simulink model "Sim_Ex33"  (R2017a)
settings: Solver=VariableStepAuto  StartTime=0.0  StopTime=Stop_Time  MaxStep=Ts  RelTol=1e-3
values from neighbouring files (symbols this model uses):
  Stop_Time = 0.12    [A_Ex33.m]
  Ts = 1/Fs    (= 5e-05)    [A_Ex33.m]
undefined symbols (not defined in the file or in its folder): DiscIntNeverNeededParam, Grid, PLL
libraries: simulink x3
settings Model: Creator=Joonhee  LastModifiedBy=Joonhee
settings SolverCC: MaxConsecutiveMinStep=1000

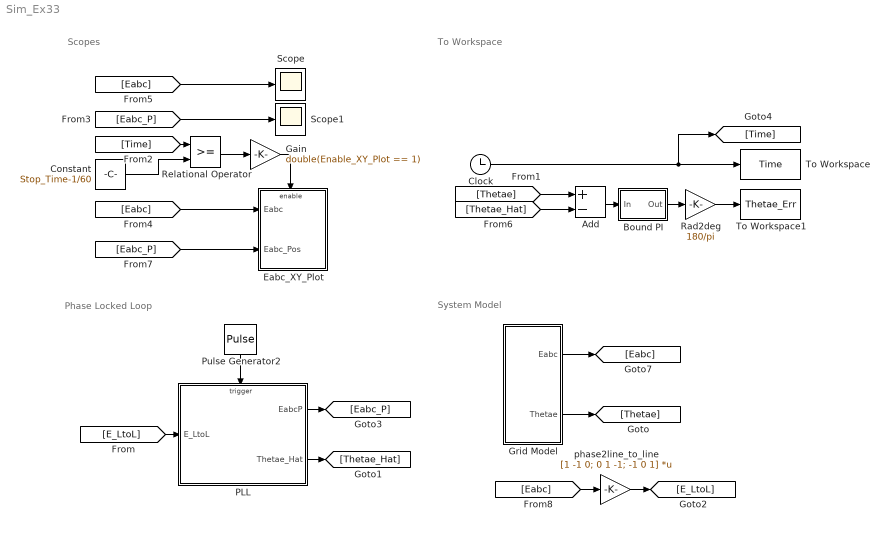
== system Sim_Ex33 ==
  note: System Model
  note: Phase Locked Loop
  note: Scopes
  note: To Workspace
  Add : Sum  Inputs=+-
  Bound PI : Subsystem
  Clock : Clock
  Constant : Constant  Value=Stop_Time-1/60
  Eabc_XY_Plot : Subsystem
  Gain : Gain  Gain=double(Enable_XY_Plot == 1)
  Grid Model : Subsystem
  PLL : Subsystem  TreatAsAtomicUnit=on
  Pulse Generator2 : DiscretePulseGenerator  PulseType=Time based  Period=Ts  PulseWidth=50
  Rad2deg : Gain  Gain=180/pi
  Relational Operator : RelationalOperator  OutDataTypeStr=boolean  RndMeth=Simplest
  Scope : Scope
  Scope1 : Scope
  To Workspace : ToWorkspace  VariableName=Time  SampleTime=Ts
  To Workspace1 : ToWorkspace  VariableName=Thetae_Err  SampleTime=Ts
  phase2line_to_line : Gain  Gain=[1 -1 0; 0 1 -1; -1 0 1]  Multiplication=Matrix(K*u)
  wires:
  Pulse Generator2/1 -> PLL/Trigger
  PLL/2(Thetae_Hat) -> [Thetae_Hat]
  PLL/1(EabcP) -> [Eabc_P]
  [E_LtoL] -> PLL/1(E_LtoL)
  Add/1 -> Bound PI/1(In)
  Bound PI/1(Out) -> Rad2deg/1
  [Thetae_Hat] -> Add/2
  Rad2deg/1 -> To Workspace1/1
  [Eabc] -> Scope/1
  [Eabc_P] -> Scope1/1
  [Thetae] -> Add/1
  Clock/1 -> To Workspace/1, [Time]
  Relational Operator/1 -> Gain/1
  [Time] -> Relational Operator/1
  Constant/1 -> Relational Operator/2
  [Eabc] -> Eabc_XY_Plot/1(Eabc)
  [Eabc_P] -> Eabc_XY_Plot/2(Eabc_Pos)
  Gain/1 -> Eabc_XY_Plot/Enable
  phase2line_to_line/1 -> [E_LtoL]
  [Eabc] -> phase2line_to_line/1
  Grid Model/2(Thetae) -> [Thetae]
  Grid Model/1(Eabc) -> [Eabc]

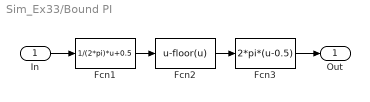
== system Sim_Ex33/Bound PI ==
  In : Inport
  Fcn1 : Fcn  Expr=1/(2*pi)*u+0.5
  Fcn2 : Fcn  Expr=u-floor(u)
  Fcn3 : Fcn  Expr=2*pi*(u-0.5)
  Out : Outport
  wires:
  Fcn1/1 -> Fcn2/1
  Fcn2/1 -> Fcn3/1
  In/1 -> Fcn1/1
  Fcn3/1 -> Out/1

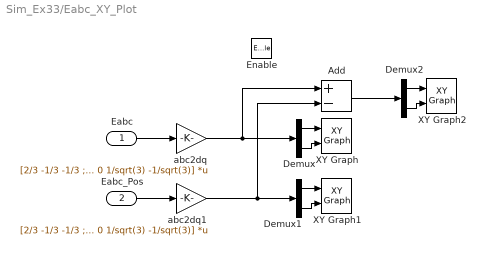
== system Sim_Ex33/Eabc_XY_Plot ==
  Eabc : Inport
  Eabc_Pos : Inport  Port=2
  Enable : EnablePort
  Add : Sum  Inputs=+-
  Demux : Demux  Outputs=2
  Demux1 : Demux  Outputs=2
  Demux2 : Demux  Outputs=2
  XY Graph : simulink/Sinks/XY Graph  xmin=-180  xmax=180  ymin=-180  ymax=180  st=-1
  XY Graph1 : simulink/Sinks/XY Graph  xmin=-180  xmax=180  ymin=-180  ymax=180  st=-1
  XY Graph2 : simulink/Sinks/XY Graph  xmin=-180  xmax=180  ymin=-180  ymax=180  st=-1
  abc2dq : Gain  Gain=[2/3 -1/3 -1/3 ; 0 1/sqrt(3) -1/sqrt(3)]  Multiplication=Matrix(K*u)  SaturateOnIntegerOverflow=on  OutDataTypeStr=Inherit: Same as input  ParamDataTypeStr=Inherit: Same as input
  abc2dq1 : Gain  Gain=[2/3 -1/3 -1/3 ; 0 1/sqrt(3) -1/sqrt(3)]  Multiplication=Matrix(K*u)  SaturateOnIntegerOverflow=on  OutDataTypeStr=Inherit: Same as input  ParamDataTypeStr=Inherit: Same as input
  wires:
  Demux/1 -> XY Graph/1
  Eabc/1 -> abc2dq/1
  Demux1/2 -> XY Graph1/2
  Demux1/1 -> XY Graph1/1
  abc2dq1/1 -> Add/2, Demux1/1
  Demux/2 -> XY Graph/2
  Eabc_Pos/1 -> abc2dq1/1
  abc2dq/1 -> Add/1, Demux/1
  Demux2/2 -> XY Graph2/2
  Demux2/1 -> XY Graph2/1
  Add/1 -> Demux2/1

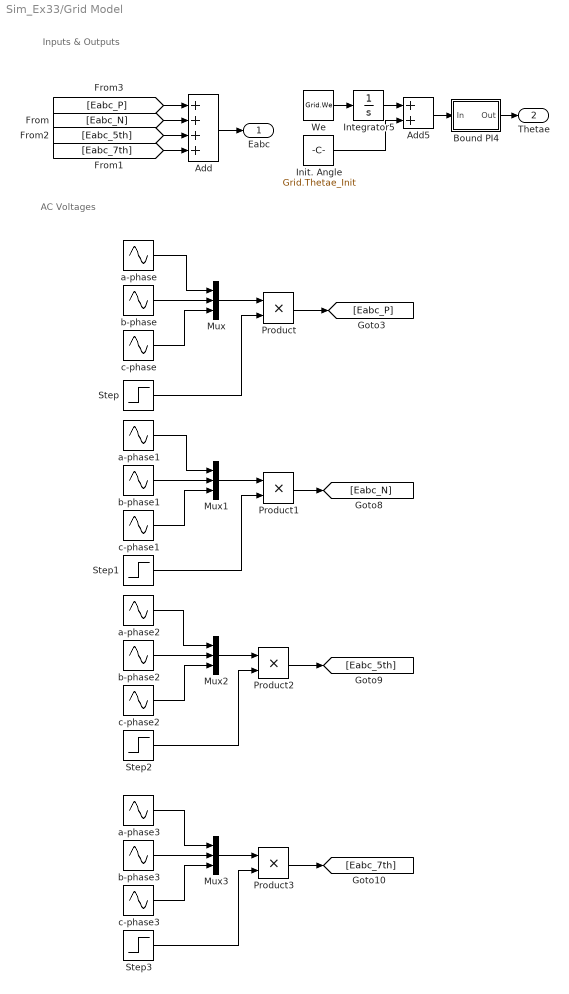
== system Sim_Ex33/Grid Model ==
  note: AC Voltages
  note: Inputs & Outputs
  Add : Sum  Inputs=++++
  Add5 : Sum
  Bound PI4 : Subsystem
  Init. Angle : Constant  Value=Grid.Thetae_Init
  Integrator5 : Integrator
  Mux{,1..3} (4 alike) : Mux  Inputs=3
  Product{,1..3} (4 alike) : Product
  Step : Step  Time=Grid.Time_Fault  Before=1  After=Grid.Ratio_P  SampleTime=0
  Step1 : Step  Time=Grid.Time_Fault  SampleTime=0
  Step2 : Step  Time=Grid.Time_Fault  SampleTime=0
  Step3 : Step  Time=Grid.Time_Fault  SampleTime=0
  We : Constant  Value=Grid.We
  a-phase : Sin  Amplitude=Grid.V_P  Frequency=Grid.We  Phase=Grid.Thetae_Init+pi  SampleTime=0
  a-phase1 : Sin  Amplitude=Grid.V_N  Frequency=Grid.We  Phase=Grid.Thetae_N_Init+pi  SampleTime=0
  a-phase2 : Sin  Amplitude=Grid.V_5th  Frequency=5*Grid.We  Phase=Grid.Thetae_5th_Init+pi  SampleTime=0
  a-phase3 : Sin  Amplitude=Grid.V_7th  Frequency=7*Grid.We  Phase=Grid.Thetae_7th_Init+pi  SampleTime=0
  b-phase : Sin  Amplitude=Grid.V_P  Frequency=Grid.We  Phase=Grid.Thetae_Init+pi-2/3*pi  SampleTime=0
  b-phase1 : Sin  Amplitude=Grid.V_N  Frequency=Grid.We  Phase=Grid.Thetae_N_Init+pi+2/3*pi  SampleTime=0
  b-phase2 : Sin  Amplitude=Grid.V_5th  Frequency=5*Grid.We  Phase=Grid.Thetae_5th_Init+pi+2/3*pi  SampleTime=0
  b-phase3 : Sin  Amplitude=Grid.V_7th  Frequency=7*Grid.We  Phase=Grid.Thetae_7th_Init+pi-2/3*pi  SampleTime=0
  c-phase : Sin  Amplitude=Grid.V_P  Frequency=Grid.We  Phase=Grid.Thetae_Init+pi-4/3*pi  SampleTime=0
  c-phase1 : Sin  Amplitude=Grid.V_N  Frequency=Grid.We  Phase=Grid.Thetae_N_Init+pi+4/3*pi  SampleTime=0
  c-phase2 : Sin  Amplitude=Grid.V_5th  Frequency=5*Grid.We  Phase=Grid.Thetae_5th_Init+pi+4/3*pi  SampleTime=0
  c-phase3 : Sin  Amplitude=Grid.V_7th  Frequency=7*Grid.We  Phase=Grid.Thetae_7th_Init+pi-4/3*pi  SampleTime=0
  Eabc : Outport
  Thetae : Outport  Port=2
  wires:
  [Eabc_P] -> Add/1
  Add/1 -> Eabc/1
  [Eabc_N] -> Add/2
  [Eabc_5th] -> Add/3
  [Eabc_7th] -> Add/4
  Bound PI4/1(Out) -> Thetae/1
  Add5/1 -> Bound PI4/1(In)
  We/1 -> Integrator5/1
  Init. Angle/1 -> Add5/2
  Integrator5/1 -> Add5/1
  b-phase/1 -> Mux/2
  a-phase/1 -> Mux/1
  c-phase/1 -> Mux/3
  c-phase1/1 -> Mux1/3
  a-phase1/1 -> Mux1/1
  b-phase1/1 -> Mux1/2
  b-phase2/1 -> Mux2/2
  a-phase2/1 -> Mux2/1
  c-phase2/1 -> Mux2/3
  c-phase3/1 -> Mux3/3
  a-phase3/1 -> Mux3/1
  b-phase3/1 -> Mux3/2
  Mux/1 -> Product/1
  Mux1/1 -> Product1/1
  Step/1 -> Product/2
  Product/1 -> [Eabc_P]
  Step1/1 -> Product1/2
  Mux2/1 -> Product2/1
  Mux3/1 -> Product3/1
  Step2/1 -> Product2/2
  Step3/1 -> Product3/2
  Product1/1 -> [Eabc_N]
  Product2/1 -> [Eabc_5th]
  Product3/1 -> [Eabc_7th]

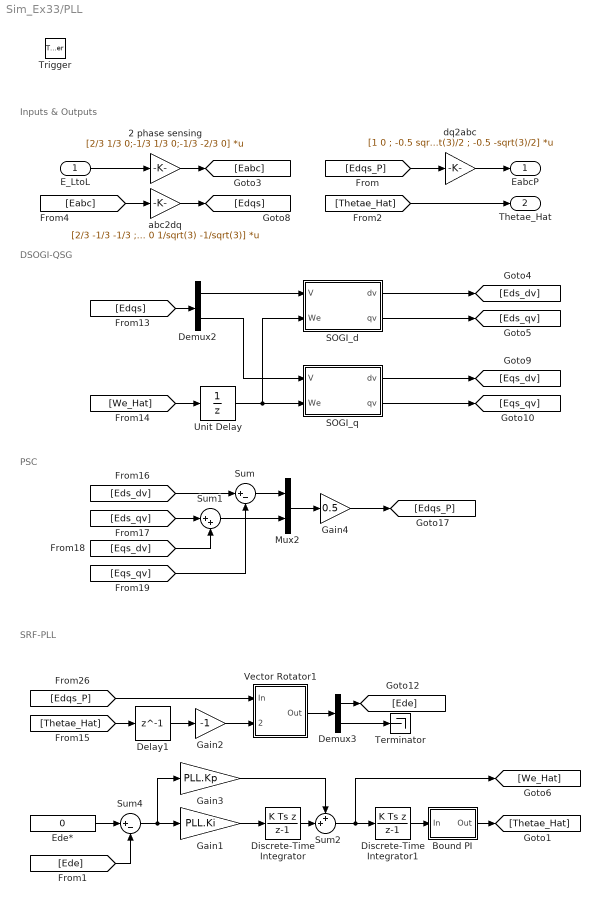
== system Sim_Ex33/PLL ==
  note: DSOGI-QSG
  note: SRF-PLL
  note: PSC
  note: Inputs & Outputs
  E_LtoL : Inport
  Trigger : TriggerPort  VariantControl=Variant
  2 phase sensing : Gain  Gain=[2/3 1/3 0;-1/3 1/3 0;-1/3 -2/3 0]  Multiplication=Matrix(K*u)  SaturateOnIntegerOverflow=on  OutDataTypeStr=Inherit: Same as input  ParamDataTypeStr=Inherit: Same as input
  Bound PI : Subsystem
  Delay1 : Delay  DelayLength=1
  Demux2 : Demux  Outputs=2
  Demux3 : Demux  Outputs=2
  Discrete-Time Integrator : DiscreteIntegrator  IntegratorMethod=Integration: Backward Euler  InitialCondition=PLL.We_FF  SampleTime=-1  ICPrevOutput=DiscIntNeverNeededParam  ICPrevScaledInput=DiscIntNeverNeededParam
  Discrete-Time Integrator1 : DiscreteIntegrator  IntegratorMethod=Integration: Backward Euler  InitialCondition=Grid.Thetae_Init+2*Grid.We*Ts  SampleTime=-1  ICPrevOutput=DiscIntNeverNeededParam  ICPrevScaledInput=DiscIntNeverNeededParam
  Ede* : Constant  Value=0
  Gain1 : Gain  Gain=PLL.Ki
  Gain2 : Gain  Gain=-1
  Gain3 : Gain  Gain=PLL.Kp
  Gain4 : Gain  Gain=0.5
  Mux2 : Mux  Inputs=2
  SOGI_d : Subsystem
  SOGI_q : Subsystem
  Sum : Sum  Inputs=|+-
  Sum1 : Sum  Inputs=|++
  Sum2 : Sum  Inputs=++|
  Sum4 : Sum  Inputs=|+-
  Terminator : Terminator
  Unit Delay : UnitDelay  SampleTime=-1
  Vector Rotator1 : Subsystem  Tag=dqs2dqw
  abc2dq : Gain  Gain=[2/3 -1/3 -1/3 ; 0 1/sqrt(3) -1/sqrt(3)]  Multiplication=Matrix(K*u)  SaturateOnIntegerOverflow=on  OutDataTypeStr=Inherit: Same as input  ParamDataTypeStr=Inherit: Same as input
  dq2abc : Gain  Gain=[1 0 ; -0.5 sqrt(3)/2 ; -0.5 -sqrt(3)/2]  Multiplication=Matrix(K*u)
  EabcP : Outport
  Thetae_Hat : Outport  Port=2
  wires:
  [Edqs_P] -> dq2abc/1
  Sum2/1 -> Discrete-Time Integrator1/1, [We_Hat]
  Discrete-Time Integrator1/1 -> Bound PI/1(In)
  Ede*/1 -> Sum4/1
  Gain1/1 -> Discrete-Time Integrator/1
  [Thetae_Hat] -> Thetae_Hat/1
  Gain4/1 -> [Edqs_P]
  SOGI_q/2(qv) -> [Eqs_qv]
  Mux2/1 -> Gain4/1
  [Eqs_dv] -> Sum1/2
  dq2abc/1 -> EabcP/1
  [We_Hat] -> Unit Delay/1
  Demux2/1 -> SOGI_d/1(V)
  [Edqs_P] -> Vector Rotator1/1(In)
  Gain2/1 -> Vector Rotator1/2(Theta)
  [Eds_qv] -> Sum1/1
  Unit Delay/1 -> SOGI_q/2(We), SOGI_d/2(We)
  [Thetae_Hat] -> Delay1/1
  Demux2/2 -> SOGI_q/1(V)
  Sum1/1 -> Mux2/2
  [Eqs_qv] -> Sum/2
  Gain3/1 -> Sum2/1
  Sum/1 -> Mux2/1
  Vector Rotator1/1(Out) -> Demux3/1
  [Eds_dv] -> Sum/1
  [Edqs] -> Demux2/1
  SOGI_d/2(qv) -> [Eds_qv]
  Bound PI/1(Out) -> [Thetae_Hat]
  Demux3/1 -> [Ede]
  Discrete-Time Integrator/1 -> Sum2/2
  SOGI_q/1(dv) -> [Eqs_dv]
  Sum4/1 -> Gain3/1, Gain1/1
  [Ede] -> Sum4/2
  Demux3/2 -> Terminator/1
  SOGI_d/1(dv) -> [Eds_dv]
  Delay1/1 -> Gain2/1
  2 phase sensing/1 -> [Eabc]
  [Eabc] -> abc2dq/1
  abc2dq/1 -> [Edqs]
  E_LtoL/1 -> 2 phase sensing/1

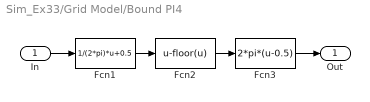
== system Sim_Ex33/Grid Model/Bound PI4 ==
  In : Inport
  Fcn1 : Fcn  Expr=1/(2*pi)*u+0.5
  Fcn2 : Fcn  Expr=u-floor(u)
  Fcn3 : Fcn  Expr=2*pi*(u-0.5)
  Out : Outport
  wires:
  Fcn1/1 -> Fcn2/1
  Fcn2/1 -> Fcn3/1
  In/1 -> Fcn1/1
  Fcn3/1 -> Out/1

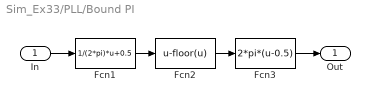
== system Sim_Ex33/PLL/Bound PI ==
  In : Inport
  Fcn1 : Fcn  Expr=1/(2*pi)*u+0.5
  Fcn2 : Fcn  Expr=u-floor(u)
  Fcn3 : Fcn  Expr=2*pi*(u-0.5)
  Out : Outport
  wires:
  Fcn1/1 -> Fcn2/1
  Fcn2/1 -> Fcn3/1
  In/1 -> Fcn1/1
  Fcn3/1 -> Out/1

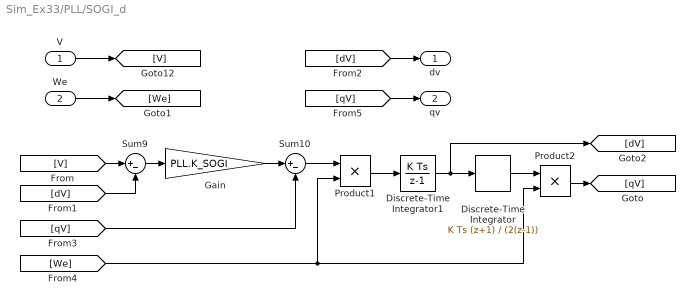
== system Sim_Ex33/PLL/SOGI_d ==
  V : Inport
  We : Inport  Port=2
  Discrete-Time Integrator : DiscreteIntegrator  IntegratorMethod=Integration: Trapezoidal  InitialCondition=Grid.V_P*cos(Grid.Thetae_Init+1.4*Grid.We*Ts)/PLL.We_FF  SampleTime=-1  ICPrevOutput=DiscIntNeverNeededParam  ICPrevScaledInput=DiscIntNeverNeededParam
  Discrete-Time Integrator1 : DiscreteIntegrator  InitialCondition=Grid.V_P*sin(Grid.Thetae_Init+pi+1.4*Grid.We*Ts)  SampleTime=-1  ICPrevOutput=DiscIntNeverNeededParam  ICPrevScaledInput=DiscIntNeverNeededParam
  Gain : Gain  Gain=PLL.K_SOGI
  Product1 : Product
  Product2 : Product
  Sum10 : Sum  Inputs=|+-
  Sum9 : Sum  Inputs=|+-
  dv : Outport
  qv : Outport  Port=2
  wires:
  [V] -> Sum9/1
  [dV] -> Sum9/2
  Sum9/1 -> Gain/1
  Gain/1 -> Sum10/1
  [qV] -> Sum10/2
  Sum10/1 -> Product1/1
  [We] -> Product1/2, Product2/2
  Product2/1 -> [qV]
  [dV] -> dv/1
  V/1 -> [V]
  We/1 -> [We]
  [qV] -> qv/1
  Product1/1 -> Discrete-Time Integrator1/1
  Discrete-Time Integrator1/1 -> [dV], Discrete-Time Integrator/1
  Discrete-Time Integrator/1 -> Product2/1

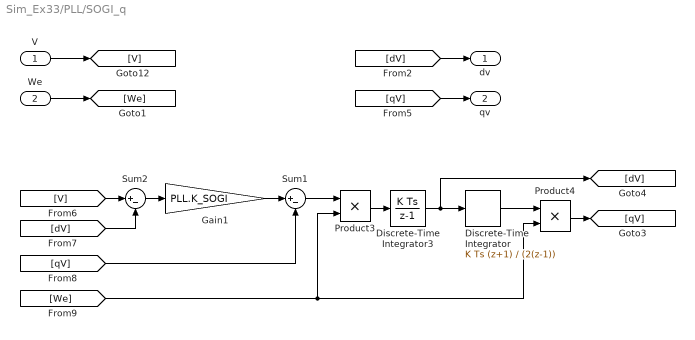
== system Sim_Ex33/PLL/SOGI_q ==
  V : Inport
  We : Inport  Port=2
  Discrete-Time Integrator : DiscreteIntegrator  IntegratorMethod=Integration: Trapezoidal  InitialCondition=Grid.V_P*sin(Grid.Thetae_Init+1.4*Grid.We*Ts)/PLL.We_FF  SampleTime=-1  ICPrevOutput=DiscIntNeverNeededParam  ICPrevScaledInput=DiscIntNeverNeededParam
  Discrete-Time Integrator3 : DiscreteIntegrator  InitialCondition=Grid.V_P*cos(Grid.Thetae_Init+1.4*Grid.We*Ts)  SampleTime=-1  ICPrevOutput=DiscIntNeverNeededParam  ICPrevScaledInput=DiscIntNeverNeededParam
  Gain1 : Gain  Gain=PLL.K_SOGI
  Product3 : Product
  Product4 : Product
  Sum1 : Sum  Inputs=|+-
  Sum2 : Sum  Inputs=|+-
  dv : Outport
  qv : Outport  Port=2
  wires:
  [qV] -> qv/1
  We/1 -> [We]
  V/1 -> [V]
  [dV] -> dv/1
  Product3/1 -> Discrete-Time Integrator3/1
  Product4/1 -> [qV]
  [We] -> Product3/2, Product4/2
  Gain1/1 -> Sum1/1
  [dV] -> Sum2/2
  Sum1/1 -> Product3/1
  [V] -> Sum2/1
  Sum2/1 -> Gain1/1
  Discrete-Time Integrator/1 -> Product4/1
  [qV] -> Sum1/2
  Discrete-Time Integrator3/1 -> [dV], Discrete-Time Integrator/1

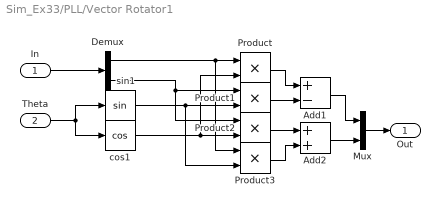
== system Sim_Ex33/PLL/Vector Rotator1 ==
  In : Inport
  Theta : Inport  Port=2
  Add1 : Sum  Inputs=+-
  Add2 : Sum
  Demux : Demux  Outputs=2
  Mux : Mux  Inputs=[1 1]
  Product{,1..3} (4 alike) : Product  RndMeth=Zero
  cos1 : Trigonometry  Operator=cos
  sin1 : Trigonometry
  Out : Outport
  wires:
  Theta/1 -> cos1/1, sin1/1
  Demux/1 -> Product3/1, Product/1
  Mux/1 -> Out/1
  In/1 -> Demux/1
  Demux/2 -> Product1/1, Product2/1
  cos1/1 -> Product/2, Product2/2
  sin1/1 -> Product1/2, Product3/2
  Product/1 -> Add1/1
  Product1/1 -> Add1/2
  Add1/1 -> Mux/1
  Product2/1 -> Add2/1
  Product3/1 -> Add2/2
  Add2/1 -> Mux/2
